simulink model "SingleTrack"  (R2019b)
settings: Solver=ode1  StartTime=0  StopTime=250  FixedStep=1.0000000000000000e-003  RelTol=1e-3
InitFcn:
  | sampleTime = str2double(get_param(bdroot, 'FixedStep'));
undefined symbols (not defined in the file or in its folder): AccPedalPos, BrakePedalPos, BrakeSwitch, DiscIntNeverNeededParam, DYNA4, EngSpd, IgnitionSwitch, InitialGear, InitialSpeed, IntendedEngTrq, LeftIndicator, MainBrakePress, MaxGear, MDL, MinGear, RefAcc, RefLane, RefLatPos, RefPath, RefPathCurv, RefSpd, RefSpdPreview, RefSpdRetrospect, RightIndicator, SteeringWheelAng, SteeringWheelTrq, UserDefinedRefValue, vm_const
libraries: UtilitiesLibrary x31, simulink x18, WheelSystemModules x13, LongitudinalControllerModules x13, LateralControllerModules x7, AnimationBusselectorModules x5, EnvironmentModules x5, BasicEngineControlModules x5, MiscellaneousControlModules x5, Animation3Modules x4, AuxiliariesModules x4, ReducedTireModules x4
(part 15 of 32)

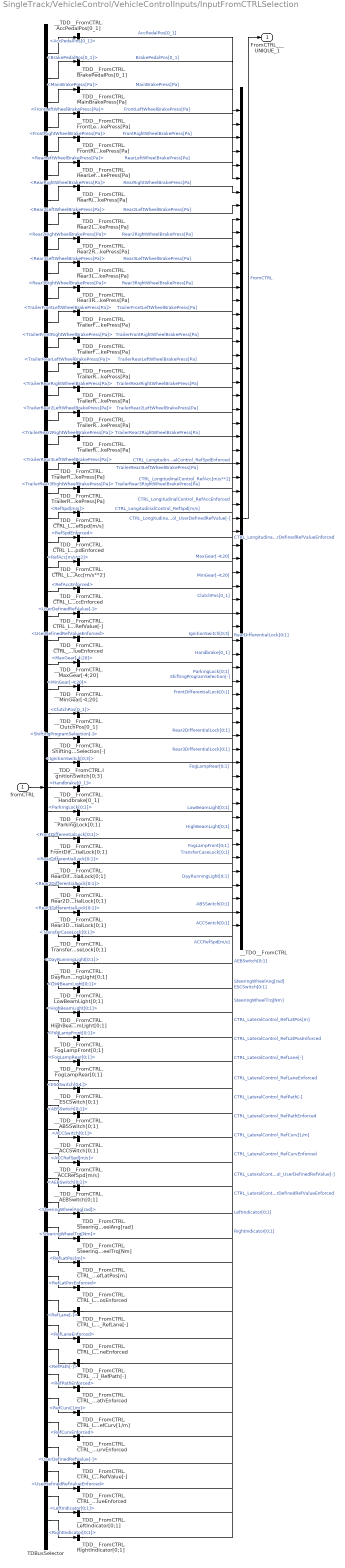
== system SingleTrack/VehicleControl/VehicleControlInputs/InputFromCTRLSelection ==
  fromCTRL : Inport
  TDBusSelector : BusSelector  OutputSignals=CTRL.LongitudinalControl.AccPedalPos[0_1],CTRL.LongitudinalControl.BrakePedalPos[0_1],CTRL.LongitudinalControl.MainBrakePress[Pa],CTRL.LongitudinalControl.FrontLeftWheelBrakePress[Pa],CTRL.LongitudinalControl.FrontRightWheelBrakePress[Pa],CTRL.LongitudinalControl.RearLeftWheelBrakePress[Pa],CTRL.LongitudinalControl.RearRightWheelBrakePress[Pa],CTRL.LongitudinalControl.Rear2LeftWheelBrakePress[Pa],CTRL.LongitudinalControl.Rear2RightWheelBrakePress[Pa],CTRL.LongitudinalControl.Rear3LeftWheelBrakePress[Pa],CTRL.LongitudinalControl.Rear3RightWheelBrakePress[Pa],CTRL.LongitudinalControl.TrailerFrontLeftWheelBrakePress[Pa],CTRL.LongitudinalControl.TrailerFrontRightWheelBrakePress[Pa],CTRL.LongitudinalControl.TrailerRearLeftWheelBrakePress[Pa],CTRL.LongitudinalControl.TrailerRearRightWheelBrakePress[Pa],CTRL.LongitudinalControl.TrailerRear2LeftWheelBrakePress[Pa],CTRL.LongitudinalControl.TrailerRear2RightWheelBrakePress[Pa],CTRL.LongitudinalControl.TrailerRear3LeftWheelBrakePress[Pa],CTRL.LongitudinalControl.TrailerRear3RightWheelBrakePress[Pa],CTRL.LongitudinalControl.RefSpd[m/s],CTRL.LongitudinalControl.RefSpdEnforced,CTRL.LongitudinalControl.RefAcc[m/s**2],CTRL.LongitudinalControl.RefAccEnforced,CTRL.LongitudinalControl.UserDefinedRefValue[-],CTRL.LongitudinalControl.UserDefinedRefValueEnforced,CTRL.LongitudinalControl.MaxGear[-4;20],CTRL.LongitudinalControl.MinGear[-4;20],CTRL.LongitudinalControl.ClutchPos[0_1],CTRL.LongitudinalControl.ShiftingProgramSelection[-],CTRL.LongitudinalControl.IgnitionSwitch[0;3],CTRL.LongitudinalControl.Handbrake[0_1],CTRL.LongitudinalControl.ParkingLock[0;1],CTRL.LongitudinalControl.FrontDifferentialLock[0;1],CTRL.LongitudinalControl.RearDifferentialLock[0;1],CTRL.LongitudinalControl.Rear2DifferentialLock[0;1],CTRL.LongitudinalControl.Rear3DifferentialLock[0;1],CTRL.LongitudinalControl.TransferCaseLock[0;1],CTRL.LongitudinalControl.DayRunningLight[0;1],CTRL.LongitudinalControl.LowBeamLight[0;1],CTRL.LongitudinalControl.HighBeamLight[0;1],CTRL.LongitudinalControl.FogLampFront[0;1],CTRL.LongitudinalControl.FogLampRear[0;1],CTRL.LongitudinalControl.ESCSwitch[0;1],CTRL.LongitudinalControl.ABSSwitch[0;1],CTRL.LongitudinalControl.ACCSwitch[0;1],CTRL.LongitudinalControl.ACCRefSpd[m/s],CTRL.LongitudinalControl.AEBSwitch[0;1],CTRL.LateralControl.SteeringWheelAng[rad],CTRL.LateralControl.SteeringWheelTrq[Nm],CTRL.LateralControl.RefLatPos[m],CTRL.LateralControl.RefLatPosEnforced,CTRL.LateralControl.RefLane[-],CTRL.LateralControl.RefLaneEnforced,CTRL.LateralControl.RefPath[-],CTRL.LateralControl.RefPathEnforced,CTRL.LateralControl.RefCurv[1/m],CTRL.LateralControl.RefCurvEnforced,CTRL.LateralControl.UserDefinedRefValue[-],CTRL.LateralControl.UserDefinedRefValueEnforced,CTRL.LateralControl.LeftIndicator[0;1],CTRL.LateralControl.RightIndicator[0;1]
  __TDD__FromCTRL.ABSSwitch[0;1] : Demux  Outputs=[1]
  __TDD__FromCTRL.ACCRefSpd[m/s] : Demux  Outputs=[1]
  __TDD__FromCTRL.ACCSwitch[0;1] : Demux  Outputs=[1]
  __TDD__FromCTRL.AEBSwitch[0;1] : Demux  Outputs=[1]
  __TDD__FromCTRL.AccPedalPos[0_1] : Demux  Outputs=[1]
  __TDD__FromCTRL.BrakePedalPos[0_1] : Demux  Outputs=[1]
  __TDD__FromCTRL.CTRL_LateralControl_RefCurvEnforced : Demux  Outputs=[1]
  __TDD__FromCTRL.CTRL_LateralControl_RefCurv[1/m] : Demux  Outputs=[1]
  __TDD__FromCTRL.CTRL_LateralControl_RefLaneEnforced : Demux  Outputs=[1]
  __TDD__FromCTRL.CTRL_LateralControl_RefLane[-] : Demux  Outputs=[1]
  __TDD__FromCTRL.CTRL_LateralControl_RefLatPosEnforced : Demux  Outputs=[1]
  __TDD__FromCTRL.CTRL_LateralControl_RefLatPos[m] : Demux  Outputs=[1]
  __TDD__FromCTRL.CTRL_LateralControl_RefPathEnforced : Demux  Outputs=[1]
  __TDD__FromCTRL.CTRL_LateralControl_RefPath[-] : Demux  Outputs=[1]
  __TDD__FromCTRL.CTRL_LateralControl_UserDefinedRefValueEnforced : Demux  Outputs=[1]
  __TDD__FromCTRL.CTRL_LateralControl_UserDefinedRefValue[-] : Demux  Outputs=[1]
  __TDD__FromCTRL.CTRL_LongitudinalControl_RefAccEnforced : Demux  Outputs=[1]
  __TDD__FromCTRL.CTRL_LongitudinalControl_RefAcc[m/s**2] : Demux  Outputs=[1]
  __TDD__FromCTRL.CTRL_LongitudinalControl_RefSpdEnforced : Demux  Outputs=[1]
  __TDD__FromCTRL.CTRL_LongitudinalControl_RefSpd[m/s] : Demux  Outputs=[1]
  __TDD__FromCTRL.CTRL_LongitudinalControl_UserDefinedRefValueEnforced : Demux  Outputs=[1]
  __TDD__FromCTRL.CTRL_LongitudinalControl_UserDefinedRefValue[-] : Demux  Outputs=[1]
  __TDD__FromCTRL.ClutchPos[0_1] : Demux  Outputs=[1]
  __TDD__FromCTRL.DayRunningLight[0;1] : Demux  Outputs=[1]
  __TDD__FromCTRL.ESCSwitch[0;1] : Demux  Outputs=[1]
  __TDD__FromCTRL.FogLampFront[0;1] : Demux  Outputs=[1]
  __TDD__FromCTRL.FogLampRear[0;1] : Demux  Outputs=[1]
  __TDD__FromCTRL.FrontDifferentialLock[0;1] : Demux  Outputs=[1]
  __TDD__FromCTRL.FrontLeftWheelBrakePress[Pa] : Demux  Outputs=[1]
  __TDD__FromCTRL.FrontRightWheelBrakePress[Pa] : Demux  Outputs=[1]
  __TDD__FromCTRL.Handbrake[0_1] : Demux  Outputs=[1]
  __TDD__FromCTRL.HighBeamLight[0;1] : Demux  Outputs=[1]
  __TDD__FromCTRL.IgnitionSwitch[0;3] : Demux  Outputs=[1]
  __TDD__FromCTRL.LeftIndicator[0;1] : Demux  Outputs=[1]
  __TDD__FromCTRL.LowBeamLight[0;1] : Demux  Outputs=[1]
  __TDD__FromCTRL.MainBrakePress[Pa] : Demux  Outputs=[1]
  __TDD__FromCTRL.MaxGear[-4;20] : Demux  Outputs=[1]
  __TDD__FromCTRL.MinGear[-4;20] : Demux  Outputs=[1]
  __TDD__FromCTRL.ParkingLock[0;1] : Demux  Outputs=[1]
  __TDD__FromCTRL.Rear2DifferentialLock[0;1] : Demux  Outputs=[1]
  __TDD__FromCTRL.Rear2LeftWheelBrakePress[Pa] : Demux  Outputs=[1]
  __TDD__FromCTRL.Rear2RightWheelBrakePress[Pa] : Demux  Outputs=[1]
  __TDD__FromCTRL.Rear3DifferentialLock[0;1] : Demux  Outputs=[1]
  __TDD__FromCTRL.Rear3LeftWheelBrakePress[Pa] : Demux  Outputs=[1]
  __TDD__FromCTRL.Rear3RightWheelBrakePress[Pa] : Demux  Outputs=[1]
  __TDD__FromCTRL.RearDifferentialLock[0;1] : Demux  Outputs=[1]
  __TDD__FromCTRL.RearLeftWheelBrakePress[Pa] : Demux  Outputs=[1]
  __TDD__FromCTRL.RearRightWheelBrakePress[Pa] : Demux  Outputs=[1]
  __TDD__FromCTRL.RightIndicator[0;1] : Demux  Outputs=[1]
  __TDD__FromCTRL.ShiftingProgramSelection[-] : Demux  Outputs=[1]
  __TDD__FromCTRL.SteeringWheelAng[rad] : Demux  Outputs=[1]
  __TDD__FromCTRL.SteeringWheelTrq[Nm] : Demux  Outputs=[1]
  __TDD__FromCTRL.TrailerFrontLeftWheelBrakePress[Pa] : Demux  Outputs=[1]
  __TDD__FromCTRL.TrailerFrontRightWheelBrakePress[Pa] : Demux  Outputs=[1]
  __TDD__FromCTRL.TrailerRear2LeftWheelBrakePress[Pa] : Demux  Outputs=[1]
  __TDD__FromCTRL.TrailerRear2RightWheelBrakePress[Pa] : Demux  Outputs=[1]
  __TDD__FromCTRL.TrailerRear3LeftWheelBrakePress[Pa] : Demux  Outputs=[1]
  __TDD__FromCTRL.TrailerRear3RightWheelBrakePress[Pa] : Demux  Outputs=[1]
  __TDD__FromCTRL.TrailerRearLeftWheelBrakePress[Pa] : Demux  Outputs=[1]
  __TDD__FromCTRL.TrailerRearRightWheelBrakePress[Pa] : Demux  Outputs=[1]
  __TDD__FromCTRL.TransferCaseLock[0;1] : Demux  Outputs=[1]
  __TDO__FromCTRL : BusCreator  Inputs=61
  FromCTRL___UNIQUE_1 : Outport  Description=|  PortDimensions=[61]  VectorParamsAs1DForOutWhenUnconnected=off
      | <name>CTRL.LongitudinalControl.AccPedalPos[0_1]</name>
      | <comment>Accelerator pedal position</comment>
  wires:
  __TDO__FromCTRL/1 -> FromCTRL___UNIQUE_1/1  "FromCTRL"
  __TDD__FromCTRL.RightIndicator[0;1]/1 -> __TDO__FromCTRL/61  "RightIndicator[0;1]"
  TDBusSelector/61 -> __TDD__FromCTRL.RightIndicator[0;1]/1  "<RightIndicator[0;1]>"
  __TDD__FromCTRL.LeftIndicator[0;1]/1 -> __TDO__FromCTRL/60  "LeftIndicator[0;1]"
  TDBusSelector/60 -> __TDD__FromCTRL.LeftIndicator[0;1]/1  "<LeftIndicator[0;1]>"
  __TDD__FromCTRL.CTRL_LateralControl_UserDefinedRefValueEnforced/1 -> __TDO__FromCTRL/59  "CTRL_LateralControl_UserDefinedRefValueEnforced"
  TDBusSelector/59 -> __TDD__FromCTRL.CTRL_LateralControl_UserDefinedRefValueEnforced/1  "<UserDefinedRefValueEnforced>"
  __TDD__FromCTRL.CTRL_LateralControl_UserDefinedRefValue[-]/1 -> __TDO__FromCTRL/58  "CTRL_LateralControl_UserDefinedRefValue[-]"
  TDBusSelector/58 -> __TDD__FromCTRL.CTRL_LateralControl_UserDefinedRefValue[-]/1  "<UserDefinedRefValue[-]>"
  __TDD__FromCTRL.CTRL_LateralControl_RefCurvEnforced/1 -> __TDO__FromCTRL/57  "CTRL_LateralControl_RefCurvEnforced"
  TDBusSelector/57 -> __TDD__FromCTRL.CTRL_LateralControl_RefCurvEnforced/1  "<RefCurvEnforced>"
  __TDD__FromCTRL.CTRL_LateralControl_RefCurv[1/m]/1 -> __TDO__FromCTRL/56  "CTRL_LateralControl_RefCurv[1/m]"
  TDBusSelector/56 -> __TDD__FromCTRL.CTRL_LateralControl_RefCurv[1/m]/1  "<RefCurv[1/m]>"
  __TDD__FromCTRL.CTRL_LateralControl_RefPathEnforced/1 -> __TDO__FromCTRL/55  "CTRL_LateralControl_RefPathEnforced"
  TDBusSelector/55 -> __TDD__FromCTRL.CTRL_LateralControl_RefPathEnforced/1  "<RefPathEnforced>"
  __TDD__FromCTRL.CTRL_LateralControl_RefPath[-]/1 -> __TDO__FromCTRL/54  "CTRL_LateralControl_RefPath[-]"
  TDBusSelector/54 -> __TDD__FromCTRL.CTRL_LateralControl_RefPath[-]/1  "<RefPath[-]>"
  __TDD__FromCTRL.CTRL_LateralControl_RefLaneEnforced/1 -> __TDO__FromCTRL/53  "CTRL_LateralControl_RefLaneEnforced"
  TDBusSelector/53 -> __TDD__FromCTRL.CTRL_LateralControl_RefLaneEnforced/1  "<RefLaneEnforced>"
  __TDD__FromCTRL.CTRL_LateralControl_RefLane[-]/1 -> __TDO__FromCTRL/52  "CTRL_LateralControl_RefLane[-]"
  TDBusSelector/52 -> __TDD__FromCTRL.CTRL_LateralControl_RefLane[-]/1  "<RefLane[-]>"
  __TDD__FromCTRL.CTRL_LateralControl_RefLatPosEnforced/1 -> __TDO__FromCTRL/51  "CTRL_LateralControl_RefLatPosEnforced"
  TDBusSelector/51 -> __TDD__FromCTRL.CTRL_LateralControl_RefLatPosEnforced/1  "<RefLatPosEnforced>"
  __TDD__FromCTRL.CTRL_LateralControl_RefLatPos[m]/1 -> __TDO__FromCTRL/50  "CTRL_LateralControl_RefLatPos[m]"
  TDBusSelector/50 -> __TDD__FromCTRL.CTRL_LateralControl_RefLatPos[m]/1  "<RefLatPos[m]>"
  __TDD__FromCTRL.SteeringWheelTrq[Nm]/1 -> __TDO__FromCTRL/49  "SteeringWheelTrq[Nm]"
  TDBusSelector/49 -> __TDD__FromCTRL.SteeringWheelTrq[Nm]/1  "<SteeringWheelTrq[Nm]>"
  __TDD__FromCTRL.SteeringWheelAng[rad]/1 -> __TDO__FromCTRL/48  "SteeringWheelAng[rad]"
  TDBusSelector/48 -> __TDD__FromCTRL.SteeringWheelAng[rad]/1  "<SteeringWheelAng[rad]>"
  __TDD__FromCTRL.AEBSwitch[0;1]/1 -> __TDO__FromCTRL/47  "AEBSwitch[0;1]"
  TDBusSelector/47 -> __TDD__FromCTRL.AEBSwitch[0;1]/1  "<AEBSwitch[0;1]>"
  __TDD__FromCTRL.ACCRefSpd[m/s]/1 -> __TDO__FromCTRL/46  "ACCRefSpd[m/s]"
  TDBusSelector/46 -> __TDD__FromCTRL.ACCRefSpd[m/s]/1  "<ACCRefSpd[m/s]>"
  __TDD__FromCTRL.ACCSwitch[0;1]/1 -> __TDO__FromCTRL/45  "ACCSwitch[0;1]"
  TDBusSelector/45 -> __TDD__FromCTRL.ACCSwitch[0;1]/1  "<ACCSwitch[0;1]>"
  __TDD__FromCTRL.ABSSwitch[0;1]/1 -> __TDO__FromCTRL/44  "ABSSwitch[0;1]"
  TDBusSelector/44 -> __TDD__FromCTRL.ABSSwitch[0;1]/1  "<ABSSwitch[0;1]>"
  __TDD__FromCTRL.ESCSwitch[0;1]/1 -> __TDO__FromCTRL/43  "ESCSwitch[0;1]"
  TDBusSelector/43 -> __TDD__FromCTRL.ESCSwitch[0;1]/1  "<ESCSwitch[0;1]>"
  __TDD__FromCTRL.FogLampRear[0;1]/1 -> __TDO__FromCTRL/42  "FogLampRear[0;1]"
  TDBusSelector/42 -> __TDD__FromCTRL.FogLampRear[0;1]/1  "<FogLampRear[0;1]>"
  __TDD__FromCTRL.FogLampFront[0;1]/1 -> __TDO__FromCTRL/41  "FogLampFront[0;1]"
  TDBusSelector/41 -> __TDD__FromCTRL.FogLampFront[0;1]/1  "<FogLampFront[0;1]>"
  __TDD__FromCTRL.HighBeamLight[0;1]/1 -> __TDO__FromCTRL/40  "HighBeamLight[0;1]"
  TDBusSelector/40 -> __TDD__FromCTRL.HighBeamLight[0;1]/1  "<HighBeamLight[0;1]>"
  __TDD__FromCTRL.LowBeamLight[0;1]/1 -> __TDO__FromCTRL/39  "LowBeamLight[0;1]"
  TDBusSelector/39 -> __TDD__FromCTRL.LowBeamLight[0;1]/1  "<LowBeamLight[0;1]>"
  __TDD__FromCTRL.DayRunningLight[0;1]/1 -> __TDO__FromCTRL/38  "DayRunningLight[0;1]"
  TDBusSelector/38 -> __TDD__FromCTRL.DayRunningLight[0;1]/1  "<DayRunningLight[0;1]>"
  __TDD__FromCTRL.TransferCaseLock[0;1]/1 -> __TDO__FromCTRL/37  "TransferCaseLock[0;1]"
  TDBusSelector/37 -> __TDD__FromCTRL.TransferCaseLock[0;1]/1  "<TransferCaseLock[0;1]>"
  __TDD__FromCTRL.Rear3DifferentialLock[0;1]/1 -> __TDO__FromCTRL/36  "Rear3DifferentialLock[0;1]"
  TDBusSelector/36 -> __TDD__FromCTRL.Rear3DifferentialLock[0;1]/1  "<Rear3DifferentialLock[0;1]>"
  __TDD__FromCTRL.Rear2DifferentialLock[0;1]/1 -> __TDO__FromCTRL/35  "Rear2DifferentialLock[0;1]"
  TDBusSelector/35 -> __TDD__FromCTRL.Rear2DifferentialLock[0;1]/1  "<Rear2DifferentialLock[0;1]>"
  __TDD__FromCTRL.RearDifferentialLock[0;1]/1 -> __TDO__FromCTRL/34  "RearDifferentialLock[0;1]"
  TDBusSelector/34 -> __TDD__FromCTRL.RearDifferentialLock[0;1]/1  "<RearDifferentialLock[0;1]>"
  __TDD__FromCTRL.FrontDifferentialLock[0;1]/1 -> __TDO__FromCTRL/33  "FrontDifferentialLock[0;1]"
  TDBusSelector/33 -> __TDD__FromCTRL.FrontDifferentialLock[0;1]/1  "<FrontDifferentialLock[0;1]>"
  __TDD__FromCTRL.ParkingLock[0;1]/1 -> __TDO__FromCTRL/32  "ParkingLock[0;1]"
  TDBusSelector/32 -> __TDD__FromCTRL.ParkingLock[0;1]/1  "<ParkingLock[0;1]>"
  __TDD__FromCTRL.Handbrake[0_1]/1 -> __TDO__FromCTRL/31  "Handbrake[0_1]"
  TDBusSelector/31 -> __TDD__FromCTRL.Handbrake[0_1]/1  "<Handbrake[0_1]>"
  __TDD__FromCTRL.IgnitionSwitch[0;3]/1 -> __TDO__FromCTRL/30  "IgnitionSwitch[0;3]"
  TDBusSelector/30 -> __TDD__FromCTRL.IgnitionSwitch[0;3]/1  "<IgnitionSwitch[0;3]>"
  __TDD__FromCTRL.ShiftingProgramSelection[-]/1 -> __TDO__FromCTRL/29  "ShiftingProgramSelection[-]"
  TDBusSelector/29 -> __TDD__FromCTRL.ShiftingProgramSelection[-]/1  "<ShiftingProgramSelection[-]>"
  __TDD__FromCTRL.ClutchPos[0_1]/1 -> __TDO__FromCTRL/28  "ClutchPos[0_1]"
  TDBusSelector/28 -> __TDD__FromCTRL.ClutchPos[0_1]/1  "<ClutchPos[0_1]>"
  __TDD__FromCTRL.MinGear[-4;20]/1 -> __TDO__FromCTRL/27  "MinGear[-4;20]"
  TDBusSelector/27 -> __TDD__FromCTRL.MinGear[-4;20]/1  "<MinGear[-4;20]>"
  __TDD__FromCTRL.MaxGear[-4;20]/1 -> __TDO__FromCTRL/26  "MaxGear[-4;20]"
  TDBusSelector/26 -> __TDD__FromCTRL.MaxGear[-4;20]/1  "<MaxGear[-4;20]>"
  __TDD__FromCTRL.CTRL_LongitudinalControl_UserDefinedRefValueEnforced/1 -> __TDO__FromCTRL/25  "CTRL_LongitudinalControl_UserDefinedRefValueEnforced"
  TDBusSelector/25 -> __TDD__FromCTRL.CTRL_LongitudinalControl_UserDefinedRefValueEnforced/1  "<UserDefinedRefValueEnforced>"
  __TDD__FromCTRL.CTRL_LongitudinalControl_UserDefinedRefValue[-]/1 -> __TDO__FromCTRL/24  "CTRL_LongitudinalControl_UserDefinedRefValue[-]"
  TDBusSelector/24 -> __TDD__FromCTRL.CTRL_LongitudinalControl_UserDefinedRefValue[-]/1  "<UserDefinedRefValue[-]>"
  __TDD__FromCTRL.CTRL_LongitudinalControl_RefAccEnforced/1 -> __TDO__FromCTRL/23  "CTRL_LongitudinalControl_RefAccEnforced"
  TDBusSelector/23 -> __TDD__FromCTRL.CTRL_LongitudinalControl_RefAccEnforced/1  "<RefAccEnforced>"
  __TDD__FromCTRL.CTRL_LongitudinalControl_RefAcc[m/s**2]/1 -> __TDO__FromCTRL/22  "CTRL_LongitudinalControl_RefAcc[m/s**2]"
  TDBusSelector/22 -> __TDD__FromCTRL.CTRL_LongitudinalControl_RefAcc[m/s**2]/1  "<RefAcc[m/s**2]>"
  __TDD__FromCTRL.CTRL_LongitudinalControl_RefSpdEnforced/1 -> __TDO__FromCTRL/21  "CTRL_LongitudinalControl_RefSpdEnforced"
  TDBusSelector/21 -> __TDD__FromCTRL.CTRL_LongitudinalControl_RefSpdEnforced/1  "<RefSpdEnforced>"
  __TDD__FromCTRL.CTRL_LongitudinalControl_RefSpd[m/s]/1 -> __TDO__FromCTRL/20  "CTRL_LongitudinalControl_RefSpd[m/s]"
  TDBusSelector/20 -> __TDD__FromCTRL.CTRL_LongitudinalControl_RefSpd[m/s]/1  "<RefSpd[m/s]>"
  __TDD__FromCTRL.TrailerRear3RightWheelBrakePress[Pa]/1 -> __TDO__FromCTRL/19  "TrailerRear3RightWheelBrakePress[Pa]"
  TDBusSelector/19 -> __TDD__FromCTRL.TrailerRear3RightWheelBrakePress[Pa]/1  "<TrailerRear3RightWheelBrakePress[Pa]>"
  __TDD__FromCTRL.TrailerRear3LeftWheelBrakePress[Pa]/1 -> __TDO__FromCTRL/18  "TrailerRear3LeftWheelBrakePress[Pa]"
  TDBusSelector/18 -> __TDD__FromCTRL.TrailerRear3LeftWheelBrakePress[Pa]/1  "<TrailerRear3LeftWheelBrakePress[Pa]>"
  __TDD__FromCTRL.TrailerRear2RightWheelBrakePress[Pa]/1 -> __TDO__FromCTRL/17  "TrailerRear2RightWheelBrakePress[Pa]"
  TDBusSelector/17 -> __TDD__FromCTRL.TrailerRear2RightWheelBrakePress[Pa]/1  "<TrailerRear2RightWheelBrakePress[Pa]>"
  __TDD__FromCTRL.TrailerRear2LeftWheelBrakePress[Pa]/1 -> __TDO__FromCTRL/16  "TrailerRear2LeftWheelBrakePress[Pa]"
  TDBusSelector/16 -> __TDD__FromCTRL.TrailerRear2LeftWheelBrakePress[Pa]/1  "<TrailerRear2LeftWheelBrakePress[Pa]>"
  __TDD__FromCTRL.TrailerRearRightWheelBrakePress[Pa]/1 -> __TDO__FromCTRL/15  "TrailerRearRightWheelBrakePress[Pa]"
  TDBusSelector/15 -> __TDD__FromCTRL.TrailerRearRightWheelBrakePress[Pa]/1  "<TrailerRearRightWheelBrakePress[Pa]>"
  __TDD__FromCTRL.TrailerRearLeftWheelBrakePress[Pa]/1 -> __TDO__FromCTRL/14  "TrailerRearLeftWheelBrakePress[Pa]"
  TDBusSelector/14 -> __TDD__FromCTRL.TrailerRearLeftWheelBrakePress[Pa]/1  "<TrailerRearLeftWheelBrakePress[Pa]>"
  __TDD__FromCTRL.TrailerFrontRightWheelBrakePress[Pa]/1 -> __TDO__FromCTRL/13  "TrailerFrontRightWheelBrakePress[Pa]"
  TDBusSelector/13 -> __TDD__FromCTRL.TrailerFrontRightWheelBrakePress[Pa]/1  "<TrailerFrontRightWheelBrakePress[Pa]>"
  __TDD__FromCTRL.TrailerFrontLeftWheelBrakePress[Pa]/1 -> __TDO__FromCTRL/12  "TrailerFrontLeftWheelBrakePress[Pa]"
  TDBusSelector/12 -> __TDD__FromCTRL.TrailerFrontLeftWheelBrakePress[Pa]/1  "<TrailerFrontLeftWheelBrakePress[Pa]>"
  __TDD__FromCTRL.Rear3RightWheelBrakePress[Pa]/1 -> __TDO__FromCTRL/11  "Rear3RightWheelBrakePress[Pa]"
  TDBusSelector/11 -> __TDD__FromCTRL.Rear3RightWheelBrakePress[Pa]/1  "<Rear3RightWheelBrakePress[Pa]>"
  __TDD__FromCTRL.Rear3LeftWheelBrakePress[Pa]/1 -> __TDO__FromCTRL/10  "Rear3LeftWheelBrakePress[Pa]"
  TDBusSelector/10 -> __TDD__FromCTRL.Rear3LeftWheelBrakePress[Pa]/1  "<Rear3LeftWheelBrakePress[Pa]>"
  __TDD__FromCTRL.Rear2RightWheelBrakePress[Pa]/1 -> __TDO__FromCTRL/9  "Rear2RightWheelBrakePress[Pa]"
  TDBusSelector/9 -> __TDD__FromCTRL.Rear2RightWheelBrakePress[Pa]/1  "<Rear2RightWheelBrakePress[Pa]>"
  __TDD__FromCTRL.Rear2LeftWheelBrakePress[Pa]/1 -> __TDO__FromCTRL/8  "Rear2LeftWheelBrakePress[Pa]"
  TDBusSelector/8 -> __TDD__FromCTRL.Rear2LeftWheelBrakePress[Pa]/1  "<Rear2LeftWheelBrakePress[Pa]>"
  __TDD__FromCTRL.RearRightWheelBrakePress[Pa]/1 -> __TDO__FromCTRL/7  "RearRightWheelBrakePress[Pa]"
  TDBusSelector/7 -> __TDD__FromCTRL.RearRightWheelBrakePress[Pa]/1  "<RearRightWheelBrakePress[Pa]>"
  __TDD__FromCTRL.RearLeftWheelBrakePress[Pa]/1 -> __TDO__FromCTRL/6  "RearLeftWheelBrakePress[Pa]"
  TDBusSelector/6 -> __TDD__FromCTRL.RearLeftWheelBrakePress[Pa]/1  "<RearLeftWheelBrakePress[Pa]>"
  __TDD__FromCTRL.FrontRightWheelBrakePress[Pa]/1 -> __TDO__FromCTRL/5  "FrontRightWheelBrakePress[Pa]"
  TDBusSelector/5 -> __TDD__FromCTRL.FrontRightWheelBrakePress[Pa]/1  "<FrontRightWheelBrakePress[Pa]>"
  __TDD__FromCTRL.FrontLeftWheelBrakePress[Pa]/1 -> __TDO__FromCTRL/4  "FrontLeftWheelBrakePress[Pa]"
  TDBusSelector/4 -> __TDD__FromCTRL.FrontLeftWheelBrakePress[Pa]/1  "<FrontLeftWheelBrakePress[Pa]>"
  __TDD__FromCTRL.MainBrakePress[Pa]/1 -> __TDO__FromCTRL/3  "MainBrakePress[Pa]"
  TDBusSelector/3 -> __TDD__FromCTRL.MainBrakePress[Pa]/1  "<MainBrakePress[Pa]>"
  __TDD__FromCTRL.BrakePedalPos[0_1]/1 -> __TDO__FromCTRL/2  "BrakePedalPos[0_1]"
  TDBusSelector/2 -> __TDD__FromCTRL.BrakePedalPos[0_1]/1  "<BrakePedalPos[0_1]>"
  __TDD__FromCTRL.AccPedalPos[0_1]/1 -> __TDO__FromCTRL/1  "AccPedalPos[0_1]"
  TDBusSelector/1 -> __TDD__FromCTRL.AccPedalPos[0_1]/1  "<AccPedalPos[0_1]>"
  fromCTRL/1 -> TDBusSelector/1

== system SingleTrack/VehicleControl/VehicleControlInputs/InputFromCTRLSelection1 ==
  fromCTRL : Inport
  TDBusSelector : BusSelector  OutputSignals=CTRL.UserDefinedPhaseTermination.UserDefinedPhaseTermination10[-],CTRL.UserDefinedPhaseTermination.UserDefinedPhaseTermination1[-],CTRL.UserDefinedPhaseTermination.UserDefinedPhaseTermination2[-],CTRL.UserDefinedPhaseTermination.UserDefinedPhaseTermination3[-],CTRL.UserDefinedPhaseTermination.UserDefinedPhaseTermination4[-],CTRL.UserDefinedPhaseTermination.UserDefinedPhaseTermination5[-],CTRL.UserDefinedPhaseTermination.UserDefinedPhaseTermination6[-],CTRL.UserDefinedPhaseTermination.UserDefinedPhaseTermination7[-],CTRL.UserDefinedPhaseTermination.UserDefinedPhaseTermination8[-],CTRL.UserDefinedPhaseTermination.UserDefinedPhaseTermination9[-]
  __TDD__UserDefinedPhaseTermination.UserDefinedPhaseTermination10[-] : Demux  Outputs=[1]
  __TDD__UserDefinedPhaseTermination.UserDefinedPhaseTermination1[-] : Demux  Outputs=[1]
  __TDD__UserDefinedPhaseTermination.UserDefinedPhaseTermination2[-] : Demux  Outputs=[1]
  __TDD__UserDefinedPhaseTermination.UserDefinedPhaseTermination3[-] : Demux  Outputs=[1]
  __TDD__UserDefinedPhaseTermination.UserDefinedPhaseTermination4[-] : Demux  Outputs=[1]
  __TDD__UserDefinedPhaseTermination.UserDefinedPhaseTermination5[-] : Demux  Outputs=[1]
  __TDD__UserDefinedPhaseTermination.UserDefinedPhaseTermination6[-] : Demux  Outputs=[1]
  __TDD__UserDefinedPhaseTermination.UserDefinedPhaseTermination7[-] : Demux  Outputs=[1]
  __TDD__UserDefinedPhaseTermination.UserDefinedPhaseTermination8[-] : Demux  Outputs=[1]
  __TDD__UserDefinedPhaseTermination.UserDefinedPhaseTermination9[-] : Demux  Outputs=[1]
  __TDO__UserDefinedPhaseTermination : BusCreator  Inputs=10
  UserDefinedPhaseTermination___UNIQUE_1 : Outport  Description=|  PortDimensions=[10]  VectorParamsAs1DForOutWhenUnconnected=off
      | <name>CTRL.UserDefinedPhaseTermination.UserDefinedPhaseTermination10[-]</name>
      | <comment></comment>
  wires:
  __TDO__UserDefinedPhaseTermination/1 -> UserDefinedPhaseTermination___UNIQUE_1/1  "UserDefinedPhaseTermination"
  __TDD__UserDefinedPhaseTermination.UserDefinedPhaseTermination9[-]/1 -> __TDO__UserDefinedPhaseTermination/10  "UserDefinedPhaseTermination9[-]"
  TDBusSelector/10 -> __TDD__UserDefinedPhaseTermination.UserDefinedPhaseTermination9[-]/1  "<UserDefinedPhaseTermination9[-]>"
  __TDD__UserDefinedPhaseTermination.UserDefinedPhaseTermination8[-]/1 -> __TDO__UserDefinedPhaseTermination/9  "UserDefinedPhaseTermination8[-]"
  TDBusSelector/9 -> __TDD__UserDefinedPhaseTermination.UserDefinedPhaseTermination8[-]/1  "<UserDefinedPhaseTermination8[-]>"
  __TDD__UserDefinedPhaseTermination.UserDefinedPhaseTermination7[-]/1 -> __TDO__UserDefinedPhaseTermination/8  "UserDefinedPhaseTermination7[-]"
  TDBusSelector/8 -> __TDD__UserDefinedPhaseTermination.UserDefinedPhaseTermination7[-]/1  "<UserDefinedPhaseTermination7[-]>"
  __TDD__UserDefinedPhaseTermination.UserDefinedPhaseTermination6[-]/1 -> __TDO__UserDefinedPhaseTermination/7  "UserDefinedPhaseTermination6[-]"
  TDBusSelector/7 -> __TDD__UserDefinedPhaseTermination.UserDefinedPhaseTermination6[-]/1  "<UserDefinedPhaseTermination6[-]>"
  __TDD__UserDefinedPhaseTermination.UserDefinedPhaseTermination5[-]/1 -> __TDO__UserDefinedPhaseTermination/6  "UserDefinedPhaseTermination5[-]"
  TDBusSelector/6 -> __TDD__UserDefinedPhaseTermination.UserDefinedPhaseTermination5[-]/1  "<UserDefinedPhaseTermination5[-]>"
  __TDD__UserDefinedPhaseTermination.UserDefinedPhaseTermination4[-]/1 -> __TDO__UserDefinedPhaseTermination/5  "UserDefinedPhaseTermination4[-]"
  TDBusSelector/5 -> __TDD__UserDefinedPhaseTermination.UserDefinedPhaseTermination4[-]/1  "<UserDefinedPhaseTermination4[-]>"
  __TDD__UserDefinedPhaseTermination.UserDefinedPhaseTermination3[-]/1 -> __TDO__UserDefinedPhaseTermination/4  "UserDefinedPhaseTermination3[-]"
  TDBusSelector/4 -> __TDD__UserDefinedPhaseTermination.UserDefinedPhaseTermination3[-]/1  "<UserDefinedPhaseTermination3[-]>"
  __TDD__UserDefinedPhaseTermination.UserDefinedPhaseTermination2[-]/1 -> __TDO__UserDefinedPhaseTermination/3  "UserDefinedPhaseTermination2[-]"
  TDBusSelector/3 -> __TDD__UserDefinedPhaseTermination.UserDefinedPhaseTermination2[-]/1  "<UserDefinedPhaseTermination2[-]>"
  __TDD__UserDefinedPhaseTermination.UserDefinedPhaseTermination1[-]/1 -> __TDO__UserDefinedPhaseTermination/2  "UserDefinedPhaseTermination1[-]"
  TDBusSelector/2 -> __TDD__UserDefinedPhaseTermination.UserDefinedPhaseTermination1[-]/1  "<UserDefinedPhaseTermination1[-]>"
  __TDD__UserDefinedPhaseTermination.UserDefinedPhaseTermination10[-]/1 -> __TDO__UserDefinedPhaseTermination/1  "UserDefinedPhaseTermination10[-]"
  TDBusSelector/1 -> __TDD__UserDefinedPhaseTermination.UserDefinedPhaseTermination10[-]/1  "<UserDefinedPhaseTermination10[-]>"
  fromCTRL/1 -> TDBusSelector/1

== system SingleTrack/VehicleControl/VehicleControlInputs/InputFromTrafficSelection ==
  fromTraffic : Inport
  TDBusSelector : BusSelector  OutputSignals=DistancesToVehicle.MyLaneFrontalDist[m],AdjacentObjectsSpeeds.MyLaneFrontalSpd[m/s]
  __TDD__FromTraffic.MyLaneFrontalDist[m] : Demux  Outputs=[1]
  __TDD__FromTraffic.MyLaneFrontalSpd[m/s] : Demux  Outputs=[1]
  __TDO__FromTraffic : BusCreator  Inputs=2
  FromTraffic___UNIQUE_1 : Outport  Description=|  PortDimensions=[2]  VectorParamsAs1DForOutWhenUnconnected=off
      | <name>DistancesToVehicle.MyLaneFrontalDist[m]</name>
      | <comment>Distance to front from next fellow car on the current lane</comment>
  wires:
  __TDO__FromTraffic/1 -> FromTraffic___UNIQUE_1/1  "FromTraffic"
  __TDD__FromTraffic.MyLaneFrontalSpd[m/s]/1 -> __TDO__FromTraffic/2  "MyLaneFrontalSpd[m/s]"
  TDBusSelector/2 -> __TDD__FromTraffic.MyLaneFrontalSpd[m/s]/1  "<MyLaneFrontalSpd[m/s]>"
  __TDD__FromTraffic.MyLaneFrontalDist[m]/1 -> __TDO__FromTraffic/1  "MyLaneFrontalDist[m]"
  TDBusSelector/1 -> __TDD__FromTraffic.MyLaneFrontalDist[m]/1  "<MyLaneFrontalDist[m]>"
  fromTraffic/1 -> TDBusSelector/1

== system SingleTrack/VehicleControl/VehicleControlInputs/InputFromTrafficSelection1 ==
  fromTraffic : Inport
  TDBusSelector : BusSelector  OutputSignals=DistancesToVehicle.LeftAdjacentLaneFrontalDist[m],DistancesToVehicle.LeftAdjacentLaneRearDist[m],DistancesToVehicle.MyLaneFrontalDist[m],DistancesToVehicle.MyLaneRearDist[m],DistancesToVehicle.RightAdjacentLaneFrontalDist[m],DistancesToVehicle.RightAdjacentLaneRearDist[m]
  __TDD__FromTraffic.LeftAdjacentLaneFrontalDist[m] : Demux  Outputs=[1]
  __TDD__FromTraffic.LeftAdjacentLaneRearDist[m] : Demux  Outputs=[1]
  __TDD__FromTraffic.MyLaneFrontalDist[m] : Demux  Outputs=[1]
  __TDD__FromTraffic.MyLaneRearDist[m] : Demux  Outputs=[1]
  __TDD__FromTraffic.RightAdjacentLaneFrontalDist[m] : Demux  Outputs=[1]
  __TDD__FromTraffic.RightAdjacentLaneRearDist[m] : Demux  Outputs=[1]
  __TDO__FromTraffic : BusCreator  Inputs=6
  FromTraffic___UNIQUE_1 : Outport  Description=|  PortDimensions=[6]  VectorParamsAs1DForOutWhenUnconnected=off
      | <name>DistancesToVehicle.LeftAdjacentLaneFrontalDist[m]</name>
      | <comment>Distance to front from next fellow car on the left adjacent lane</comment>
  wires:
  __TDO__FromTraffic/1 -> FromTraffic___UNIQUE_1/1  "FromTraffic"
  __TDD__FromTraffic.RightAdjacentLaneRearDist[m]/1 -> __TDO__FromTraffic/6  "RightAdjacentLaneRearDist[m]"
  TDBusSelector/6 -> __TDD__FromTraffic.RightAdjacentLaneRearDist[m]/1  "<RightAdjacentLaneRearDist[m]>"
  __TDD__FromTraffic.RightAdjacentLaneFrontalDist[m]/1 -> __TDO__FromTraffic/5  "RightAdjacentLaneFrontalDist[m]"
  TDBusSelector/5 -> __TDD__FromTraffic.RightAdjacentLaneFrontalDist[m]/1  "<RightAdjacentLaneFrontalDist[m]>"
  __TDD__FromTraffic.MyLaneRearDist[m]/1 -> __TDO__FromTraffic/4  "MyLaneRearDist[m]"
  TDBusSelector/4 -> __TDD__FromTraffic.MyLaneRearDist[m]/1  "<MyLaneRearDist[m]>"
  __TDD__FromTraffic.MyLaneFrontalDist[m]/1 -> __TDO__FromTraffic/3  "MyLaneFrontalDist[m]"
  TDBusSelector/3 -> __TDD__FromTraffic.MyLaneFrontalDist[m]/1  "<MyLaneFrontalDist[m]>"
  __TDD__FromTraffic.LeftAdjacentLaneRearDist[m]/1 -> __TDO__FromTraffic/2  "LeftAdjacentLaneRearDist[m]"
  TDBusSelector/2 -> __TDD__FromTraffic.LeftAdjacentLaneRearDist[m]/1  "<LeftAdjacentLaneRearDist[m]>"
  __TDD__FromTraffic.LeftAdjacentLaneFrontalDist[m]/1 -> __TDO__FromTraffic/1  "LeftAdjacentLaneFrontalDist[m]"
  TDBusSelector/1 -> __TDD__FromTraffic.LeftAdjacentLaneFrontalDist[m]/1  "<LeftAdjacentLaneFrontalDist[m]>"
  fromTraffic/1 -> TDBusSelector/1

== system SingleTrack/VehicleControl/VehicleControlInputs/InputFromTrailerSelection ==
  fromTrailer : Inport
  TDBusSelector : BusSelector  OutputSignals=TrailerDriverInfo.OverallMass[kg],TrailerDriverInfo.SumWheelRotAxisInrt[kg*m**2],TrailerDriverInfo.SumMaxRollingResistanceTrq[Nm]
  __TDD__FromTrailer.OverallMass[kg] : Demux  Outputs=[1]
  __TDD__FromTrailer.SumMaxRollingResistanceTrq[Nm] : Demux  Outputs=[1]
  __TDD__FromTrailer.SumWheelRotAxisInrt[kg*m**2] : Demux  Outputs=[1]
  __TDO__FromTrailer : BusCreator  Inputs=3
  FromTrailer___UNIQUE_1 : Outport  Description=|  PortDimensions=[3]  VectorParamsAs1DForOutWhenUnconnected=off
      | <name>TrailerDriverInfo.OverallMass[kg]</name>
      | <comment></comment>
  wires:
  __TDO__FromTrailer/1 -> FromTrailer___UNIQUE_1/1  "FromTrailer"
  __TDD__FromTrailer.SumMaxRollingResistanceTrq[Nm]/1 -> __TDO__FromTrailer/3  "SumMaxRollingResistanceTrq[Nm]"
  TDBusSelector/3 -> __TDD__FromTrailer.SumMaxRollingResistanceTrq[Nm]/1  "<SumMaxRollingResistanceTrq[Nm]>"
  __TDD__FromTrailer.SumWheelRotAxisInrt[kg*m**2]/1 -> __TDO__FromTrailer/2  "SumWheelRotAxisInrt[kg*m**2]"
  TDBusSelector/2 -> __TDD__FromTrailer.SumWheelRotAxisInrt[kg*m**2]/1  "<SumWheelRotAxisInrt[kg*m**2]>"
  __TDD__FromTrailer.OverallMass[kg]/1 -> __TDO__FromTrailer/1  "OverallMass[kg]"
  TDBusSelector/1 -> __TDD__FromTrailer.OverallMass[kg]/1  "<OverallMass[kg]>"
  fromTrailer/1 -> TDBusSelector/1
